simulink subsystem "PID_Ideal"  (R2022b)
settings: Solver=VariableStepAuto  StartTime=0.0  StopTime=10.0  RelTol=1e-3
model mask{Kp=10, Ki=0.01, Kd=100e-6}
  mask prompts: Kp "Propotional"; Ki "Integral"; Kd "Drevative"
settings Model: Creator=MAAM  LastModifiedBy=MAAM

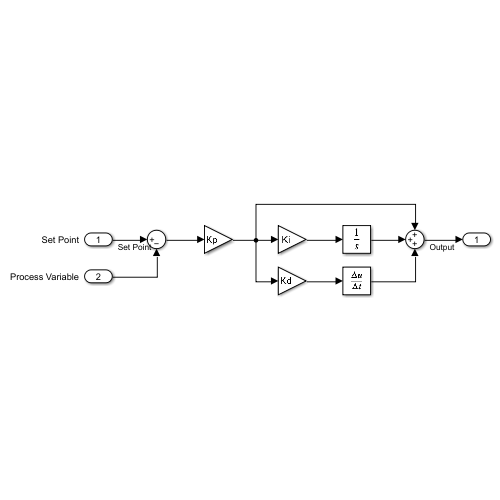
[thumbnail: Simulink's stored preview of the top-level diagram]
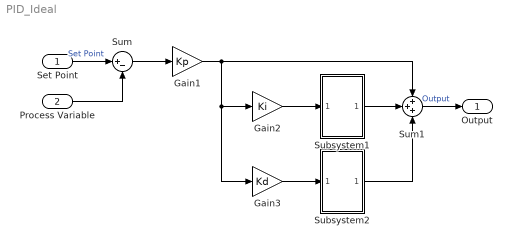
== system PID_Ideal ==
  Set Point : Inport
  Process Variable : Inport  Port=2
  Gain1 : Gain  Gain=Kp
  Gain2 : Gain  Gain=Ki
  Gain3 : Gain  Gain=Kd
  Subsystem1 : Subsystem  ReferencedSubsystem=Integrator  Gain=1.0  Init=0  SampleTime=-1  Ts=0.001
  Subsystem2 : Subsystem  ReferencedSubsystem=Derivative  Gain=1.0  Init=0  SampleTime=-1  Ts=0.001
  Sum : Sum  Inputs=|+-
  Sum1 : Sum  Inputs=+++
  Output : Outport
  wires:
  Set Point/1 -> Sum/1  "Set Point"
  Gain3/1 -> Subsystem2/1
  Gain1/1 -> Sum1/1, Gain3/1, Gain2/1
  Process Variable/1 -> Sum/2
  Sum/1 -> Gain1/1
  Gain2/1 -> Subsystem1/1
  Subsystem1/1 -> Sum1/2
  Subsystem2/1 -> Sum1/3
  Sum1/1 -> Output/1  "Output"
